simulink model "chaser_target_slosh"  (R2024a)
settings: Solver=VariableStepAuto  StartTime=0.0  StopTime=10.0  RelTol=1e-3
values from neighbouring files (symbols this model uses):
  dispslosh = 0.2    [main.m]
undefined symbols (not defined in the file or in its folder): chaser, InvDyn, KIN, reaction_wheels, slosh, solar_panel_big_reduced_FEM, solar_panel_target_reduced_FEM, target, ureal, uss, wn_big, wn_target
libraries: RCTblocks x54, SDTlibV1 x44
(part 1 of 3)
settings Model: Creator=T.FORMOSA  LastModifiedBy=r.de-oliveira
settings SolverCC: AlgebraicLoopSolver=TrustRegion
settings DebuggingCC: AlgebraicLoopMsg=none  UnconnectedInputMsg=warning  UnconnectedOutputMsg=warning  UnconnectedLineMsg=warning  ArithmeticOperatorsInVariantConditions=warning
settings ModelReferenceCC: EnableRefExpFcnMdlSchedulingChecks=on
settings SFSimCC: CustomCodeUndefinedFunction=UseInterfaceOnly
settings RTWCC: GPUComputeCapability=3.5  DLArmComputeVersion=19.05

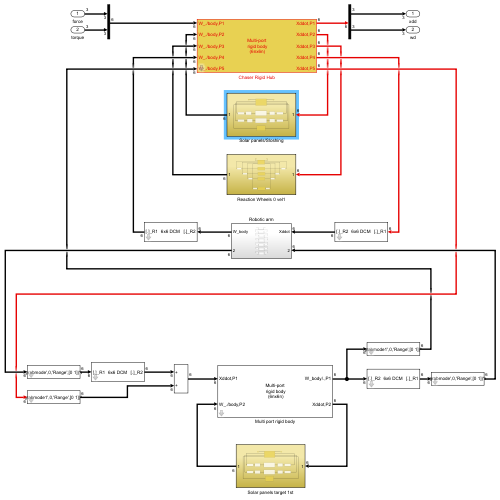
[thumbnail: Simulink's stored preview of the top-level diagram]
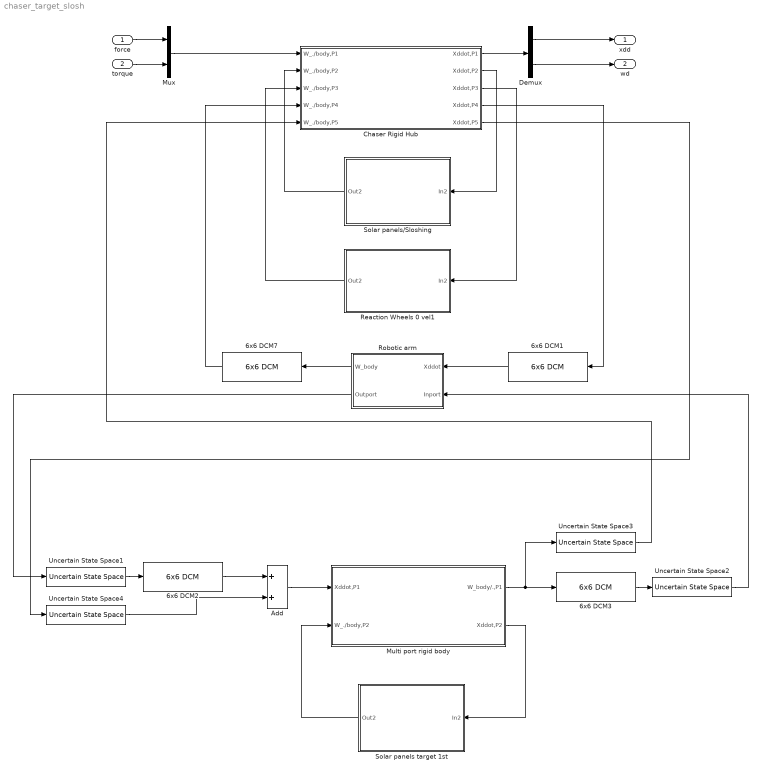
== system chaser_target_slosh ==
  force : Inport
  torque : Inport  Port=2
  6x6 DCM1 : SDTlibV1/3//6 dof DCM/6x6 DCM  rot=[-1 0 0;0 1 0;0 0 -1]  transp=on
      settings: SourceProductName=SDTlib
  6x6 DCM2 : SDTlibV1/3//6 dof DCM/6x6 DCM  rot=[0 1 0;1 0 0;0 0 -1]  transp=on
      settings: SourceProductName=SDTlib
  6x6 DCM3 : SDTlibV1/3//6 dof DCM/6x6 DCM  rot=[0 1 0;1 0 0;0 0 -1]  transp=off
      settings: SourceProductName=SDTlib
  6x6 DCM7 : SDTlibV1/3//6 dof DCM/6x6 DCM  rot=[-1 0 0;0 1 0;0 0 -1]  transp=off
      settings: SourceProductName=SDTlib
  Add : Sum
  Chaser Rigid Hub : Subsystem  mask(Multi-port rigid body (6nx6n)){m=chaser.rigidhub.wetmass, Ig=chaser.rigidhub.inertias, OG=[0;0;0], n=5, numinv=none, OP1=[0;0;0], OP2=[0;0;0], OP3=[0;0;0], OP4=[chaser.rigidhub.length/2*1.37;0;-chaser.rigidhub.height/2-0.01/2], OP5=[-1.8503e-1;-1.37618e-10;-6.3520e-1]}
      mask prompts: m "Mass (Kg)"; Ig "Inertia (at G, Kg m^2)"; OG "OG (3x1 vector, m)"; n "Number of ports"; numinv "Port to be inverted"; OP1 "OP1 (3x1 vector, m)"; OP2 "OP2 (3x1 vector, m)"; OP3 "OP3 (3x1 vector, m)"; OP4 "OP4 (3x1 vector, m)"; OP5 "OP5 (3x1 vector,m)"
      mask help:
      | 6nx6n inverse dynamic model between:
      |    *  wrenches applied to this body at the given n points,
      |    * acceleration twiists at he n given points.
      |
      | The 6x6 channel asociated to a single given point can be inverted
      mask init:
      | MultiPortRigidBody
      mask Help: web('Docmultiportrigidbody.html')
      mask TypeOptions n: 1 | 2 | 3 | 4 | 5
      mask TypeOptions numinv: none | 1 | 2 | 3 | 4 | 5
      mask DialogControl Control1 Prompt: Inverse Dynamic model of a rigid body at n given points (ports):
      mask DialogControl Control2 Prompt: 6nx6n transfer between wrenches applied at the n points and accelaretion twists at these points
      mask DialogControl Control3 Prompt: 0: the reference point
      mask DialogControl Control4 Prompt: G: the center of mass
      mask DialogControl Control5 Prompt: Pi (i=1:n): the n given connection points (n<6).
      mask DialogControl Control6 Prompt: All parameters are expressed in the body frame.
      mask DialogControl Control7 Prompt: Each parameter can be an uncertain parameter declared with "ureal"
      mask DialogControl Control8 Prompt: The 6x6 channel associated to one port can be inverted: then the input of this channel is the acceleration twist imposed at this point and the output is the wrench applied by this body.
      mask DialogControl ParameterGroupVar Prompt: Main parameters
      mask DialogControl port1 Prompt: Port #1
      mask DialogControl port2 Prompt: #2
      mask DialogControl port3 Prompt: #3
      mask DialogControl port4 Prompt: #4
      mask DialogControl port5 Prompt: #5
      mask Display:
      | disp('Multi-port\n rigid body\n (6nx6n)')
      | if n==1,
      |     if numinv-1==1,
      |         port_label('input', 1,'Xddot,P')
      |         port_label('output',1,'W_body/.,P')
      |     else
      |         port_label('input', 1,'W_./body,P')
      |         port_label('output',1,'Xddot,P')
      |     end
      | else
      |     for ii=1:n
      |         if numinv==ii+1,
      |             port_label('output',ii,['W_body/.,P',num2str(ii)])
      |             port_label('input', ii,['Xddot,P',num2str(ii)])
      |         else
      |             port_label('input', ii,['W_./body,P',num2str(ii)])
      |             port_label('output',ii,['Xddot,P',num2str(ii)])
      |         end
      |     end
      | end
  Demux : Demux  Outputs=[3 3]
  Multi port rigid body : Subsystem  mask(Multi-port rigid body (6nx6n)){m=target.rigidhub.wetmass_SDT, Ig=target.rigidhub.inertias_SDT, OG=[0;0;0], n=2, numinv=1, OP1=[-chaser.rigidhub.length*0.7/2;0;0]*ureal('grabmode',0,'Range',[0 1]), OP2=[0;0;0], OP3=[ureal('P3_y',1,'percent',10);0;0], OP4=[0;0;0], OP5=[0;0;0]}
      mask prompts: m "Mass (Kg)"; Ig "Inertia (at G, Kg m^2)"; OG "OG (3x1 vector, m)"; n "Number of ports"; numinv "Port to be inverted"; OP1 "OP1 (3x1 vector, m)"; OP2 "OP2 (3x1 vector, m)"; OP3 "OP3 (3x1 vector, m)"; OP4 "OP4 (3x1 vector, m)"; OP5 "OP5 (3x1 vector,m)"
      mask help:
      | 6nx6n dynamic model of a rigid body at n given points (ports) between wrenches applied at the n points (input) and acceleration twists at these points (output).
      |
      | 0: the reference point
      | G: the center of mass
      | Pi (i=1:n): the n given connection points (n<6).
      |
      | All parameters are expressed in the body frame.
      | Each parameter can be an uncertain parameter declared with "ureal"
      |
      | The 6x6 channel associated to one port can be inverted: then the input of this channel is the acceleration twist imposed at this point and the output is the wrench applied by this body.
      mask init:
      | MultiPortRigidBody
      mask Help: web('Docmultiportrigidbody.html')
      mask TypeOptions n: 1 | 2 | 3 | 4 | 5
      mask TypeOptions numinv: none | 1 | 2 | 3 | 4 | 5
      mask DialogControl ParameterGroupVar Prompt: Main parameters
      mask DialogControl port1 Prompt: Port #1
      mask DialogControl port2 Prompt: #2
      mask DialogControl port3 Prompt: #3
      mask DialogControl port4 Prompt: #4
      mask DialogControl port5 Prompt: #5
      mask Display:
      | disp('Multi-port\n rigid body\n (6nx6n)')
      | if n==1,
      |     if numinv-1==1,
      |         port_label('input', 1,'Xddot,P')
      |         port_label('output',1,'W_body/.,P')
      |     else
      |         port_label('input', 1,'W_./body,P')
      |         port_label('output',1,'Xddot,P')
      |     end
      | else
      |     for ii=1:n
      |         if numinv==ii+1,
      |             port_label('output',ii,['W_body/.,P',num2str(ii)])
      |             port_label('input', ii,['Xddot,P',num2str(ii)])
      |         else
      |             port_label('input', ii,['W_./body,P',num2str(ii)])
      |             port_label('output',ii,['Xddot,P',num2str(ii)])
      |         end
      |     end
      | end
  Mux : Mux  Inputs=[3 3]
  Reaction Wheels 0 vel1 : Subsystem
  Robotic arm : Subsystem
  Solar panels target 1st : Subsystem
  Solar panels/Sloshing : Subsystem
  Uncertain State Space1 : RCTblocks/Uncertain State Space  Tag=USS  USystem=ureal('grabmode',0,'Range',[0 1])*eye(6)  UValue=[]  X0=[]  uX0=[]
  Uncertain State Space2 : RCTblocks/Uncertain State Space  Tag=USS  USystem=ureal('grabmode',0,'Range',[0 1])*eye(6)  UValue=[]  X0=[]  uX0=[]
  Uncertain State Space3 : RCTblocks/Uncertain State Space  Tag=USS  USystem=ureal('grabmode1',0,'Range',[0 1])*eye(6)  UValue=[]  X0=[]  uX0=[]
  Uncertain State Space4 : RCTblocks/Uncertain State Space  Tag=USS  USystem=ureal('grabmode1',0,'Range',[0 1])*eye(6)  UValue=[]  X0=[]  uX0=[]
  xdd : Outport
  wd : Outport  Port=2
  wires:
  Reaction Wheels 0 vel1/1(Out2) -> Chaser Rigid Hub/3(W_./body,P3)
  Solar panels/Sloshing/1(Out2) -> Chaser Rigid Hub/2(W_./body,P2)
  Chaser Rigid Hub/1(Xddot,P1) -> Demux/1
  torque/1 -> Mux/2
  force/1 -> Mux/1
  Demux/1 -> xdd/1
  Chaser Rigid Hub/2(Xddot,P2) -> Solar panels/Sloshing/1(In2)
  Robotic arm/1(W_body) -> 6x6 DCM7/1
  6x6 DCM1/1 -> Robotic arm/1(Xddot)
  6x6 DCM7/1 -> Chaser Rigid Hub/4(W_./body,P4)
  6x6 DCM3/1 -> Uncertain State Space2/1
  Uncertain State Space1/1 -> 6x6 DCM2/1
  Uncertain State Space4/1 -> Add/2
  Add/1 -> Multi port rigid body/1(Xddot,P1)
  Multi port rigid body/2(Xddot,P2) -> Solar panels target 1st/1(In2)
  Solar panels target 1st/1(Out2) -> Multi port rigid body/2(W_./body,P2)
  6x6 DCM2/1 -> Add/1
  Chaser Rigid Hub/3(Xddot,P3) -> Reaction Wheels 0 vel1/1(In2)
  Chaser Rigid Hub/4(Xddot,P4) -> 6x6 DCM1/1
  Chaser Rigid Hub/5(Xddot,P5) -> Uncertain State Space4/1
  Uncertain State Space3/1 -> Chaser Rigid Hub/5(W_./body,P5)
  Robotic arm/2(Outport) -> Uncertain State Space1/1
  Uncertain State Space2/1 -> Robotic arm/2(Inport)
  Mux/1 -> Chaser Rigid Hub/1(W_./body,P1)
  Demux/2 -> wd/1
  Multi port rigid body/1(W_body/.,P1) -> Uncertain State Space3/1, 6x6 DCM3/1

== system chaser_target_slosh/Chaser Rigid Hub ==
  W_./body,P1 : Inport  PortDimensions=6
  W_./body,P2 : Inport  Port=2  PortDimensions=6
  W_./body,P3 : Inport  Port=3  PortDimensions=6
  W_./body,P4 : Inport  Port=4  PortDimensions=6
  W_./body,P5 : Inport  Port=5  PortDimensions=6
  Demux : Demux  Outputs=[6 6 6 6 6]
  Gain : RCTblocks/Uncertain State Space  Tag=USS  USystem=uss(InvDyn)  UValue=[]  X0=[]  uX0=[]
  Mux : Mux  Inputs=[6 6 6 6 6]
  Xddot,P1 : Outport
  Xddot,P2 : Outport  Port=2
  Xddot,P3 : Outport  Port=3
  Xddot,P4 : Outport  Port=4
  Xddot,P5 : Outport  Port=5
  wires:
  Mux/1 -> Gain/1
  Gain/1 -> Demux/1
  W_./body,P1/1 -> Mux/1
  Demux/1 -> Xddot,P1/1
  W_./body,P2/1 -> Mux/2
  Demux/2 -> Xddot,P2/1
  W_./body,P3/1 -> Mux/3
  Demux/3 -> Xddot,P3/1
  W_./body,P4/1 -> Mux/4
  Demux/4 -> Xddot,P4/1
  W_./body,P5/1 -> Mux/5
  Demux/5 -> Xddot,P5/1

== system chaser_target_slosh/Multi port rigid body ==
  Xddot,P1 : Inport  PortDimensions=6
  W_./body,P2 : Inport  Port=2  PortDimensions=6
  Demux : Demux  Outputs=[6 6]
  Gain : RCTblocks/Uncertain State Space  Tag=USS  USystem=uss(InvDyn)  UValue=[]  X0=[]  uX0=[]
  Mux : Mux  Inputs=[6 6]
  W_body/.,P1 : Outport
  Xddot,P2 : Outport  Port=2
  wires:
  Mux/1 -> Gain/1
  Gain/1 -> Demux/1
  Xddot,P1/1 -> Mux/1
  Demux/1 -> W_body/.,P1/1
  W_./body,P2/1 -> Mux/2
  Demux/2 -> Xddot,P2/1

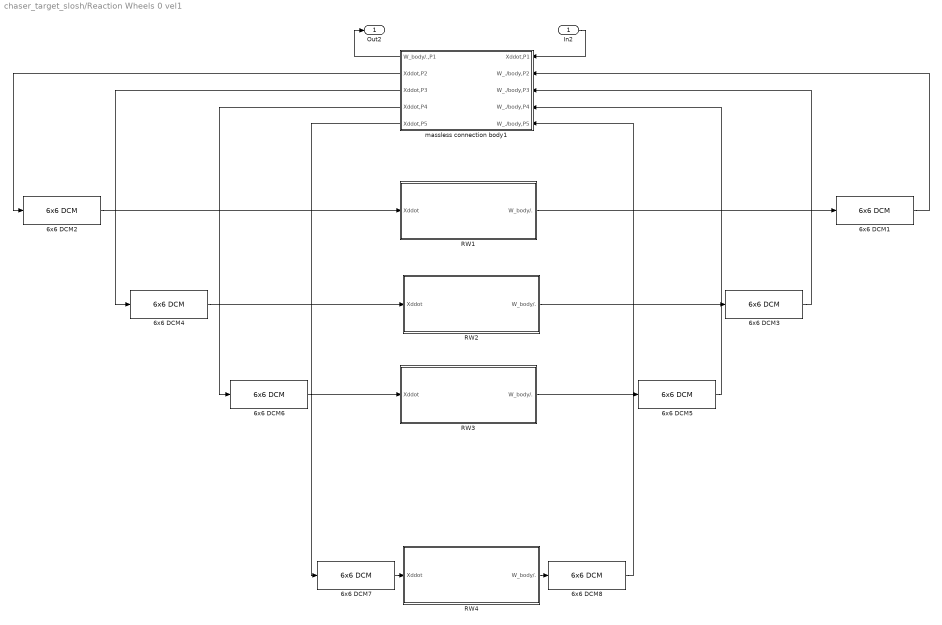
== system chaser_target_slosh/Reaction Wheels 0 vel1 ==
  In2 : Inport
  6x6 DCM1 : SDTlibV1/3//6 dof DCM/6x6 DCM  rot=chaser.GNC.control.reaction_wheels.DCM(:, :, 1)  transp=off
      settings: SourceProductName=SDTlib
  6x6 DCM2 : SDTlibV1/3//6 dof DCM/6x6 DCM  rot=chaser.GNC.control.reaction_wheels.DCM(:, :, 1)  transp=on
      settings: SourceProductName=SDTlib
  6x6 DCM3 : SDTlibV1/3//6 dof DCM/6x6 DCM  rot=chaser.GNC.control.reaction_wheels.DCM(:, :, 2)  transp=off
      settings: SourceProductName=SDTlib
  6x6 DCM4 : SDTlibV1/3//6 dof DCM/6x6 DCM  rot=chaser.GNC.control.reaction_wheels.DCM(:, :, 2)  transp=on
      settings: SourceProductName=SDTlib
  6x6 DCM5 : SDTlibV1/3//6 dof DCM/6x6 DCM  rot=chaser.GNC.control.reaction_wheels.DCM(:, :, 3)  transp=off
      settings: SourceProductName=SDTlib
  6x6 DCM6 : SDTlibV1/3//6 dof DCM/6x6 DCM  rot=chaser.GNC.control.reaction_wheels.DCM(:, :, 3)  transp=on
      settings: SourceProductName=SDTlib
  6x6 DCM7 : SDTlibV1/3//6 dof DCM/6x6 DCM  rot=chaser.GNC.control.reaction_wheels.DCM(:, :, 4)  transp=on
      settings: SourceProductName=SDTlib
  6x6 DCM8 : SDTlibV1/3//6 dof DCM/6x6 DCM  rot=chaser.GNC.control.reaction_wheels.DCM(:, :, 4)  transp=off
      settings: SourceProductName=SDTlib
  RW1 : Subsystem  AncestorBlock=SDTlibV1/6 dof bodies/1 port spinning wheel  mask(One-port spinning wheel (6x6)){ra=[0;0;1], m=chaser.reactionwheels.mass, Iw=chaser.reactionwheels.axialinertia, Ir=chaser.reactionwheels.radialinertia, OG=[0;0;0], OP=[0;0;0], Omega=reaction_wheels.initial_w_SDT(1)}
      mask prompts: ra "Wheel axis (3x1 vector)"; m "Wheel mass (Kg)"; Iw "Wheel axial Inertia  (at G, Kgm^2)"; Ir "Wheel radial inertia (at G, Kgm^2)"; OG "OG (3x1 vector, m)"; OP "OP (3x1 vector, m)"; Omega "spinning rate (rd/s)"
      mask help:
      | Dynamic model of an onboard angular momentum (spinning wheel) at point P (connection point with a parent body):
      | 6x6 transfer between accelaretion twist at P and wrench applied by this body at P.
      | 0: the reference point
      | G: the center of the wheel
      | P: the connection point
      |
      | All parameters are expressed in the (inherit) body frame.
      | Only the spinning rate can be an uncertain parameter declared with "ureal"
      mask init:
      | pass=ra2DCMi(ra);
      | Tau_GP=kinematic_model(OG,OP);
      mask Help: web('DocMomentum.html')
      mask DialogControl ParameterGroupVar Prompt: Main parameters
      mask Display:
      | disp('One-port\n angular momemtum\n (6x6)')
      | port_label('input', 1, 'Xddot')
      | port_label('output', 1, 'W_body/.')
  RW2 : Subsystem  AncestorBlock=SDTlibV1/6 dof bodies/1 port spinning wheel  mask(One-port spinning wheel (6x6)){ra=[0;0;1], m=chaser.reactionwheels.mass, Iw=chaser.reactionwheels.axialinertia, Ir=chaser.reactionwheels.radialinertia, OG=[0;0;0], OP=[0;0;0], Omega=reaction_wheels.initial_w_SDT(2)}
      mask prompts: ra "Wheel axis (3x1 vector)"; m "Wheel mass (Kg)"; Iw "Wheel axial Inertia  (at G, Kgm^2)"; Ir "Wheel radial inertia (at G, Kgm^2)"; OG "OG (3x1 vector, m)"; OP "OP (3x1 vector, m)"; Omega "spinning rate (rd/s)"
      mask help:
      | Dynamic model of an onboard angular momentum (spinning wheel) at point P (connection point with a parent body):
      | 6x6 transfer between accelaretion twist at P and wrench applied by this body at P.
      | 0: the reference point
      | G: the center of the wheel
      | P: the connection point
      |
      | All parameters are expressed in the (inherit) body frame.
      | Only the spinning rate can be an uncertain parameter declared with "ureal"
      mask init:
      | pass=ra2DCMi(ra);
      | Tau_GP=kinematic_model(OG,OP);
      mask Help: web('DocMomentum.html')
      mask DialogControl ParameterGroupVar Prompt: Main parameters
      mask Display:
      | disp('One-port\n angular momemtum\n (6x6)')
      | port_label('input', 1, 'Xddot')
      | port_label('output', 1, 'W_body/.')
  RW3 : Subsystem  AncestorBlock=SDTlibV1/6 dof bodies/1 port spinning wheel  mask(One-port spinning wheel (6x6)){ra=[0;0;1], m=chaser.reactionwheels.mass, Iw=chaser.reactionwheels.axialinertia, Ir=chaser.reactionwheels.radialinertia, OG=[0;0;0], OP=[0;0;0], Omega=reaction_wheels.initial_w_SDT(3)}
      mask prompts: ra "Wheel axis (3x1 vector)"; m "Wheel mass (Kg)"; Iw "Wheel axial Inertia  (at G, Kgm^2)"; Ir "Wheel radial inertia (at G, Kgm^2)"; OG "OG (3x1 vector, m)"; OP "OP (3x1 vector, m)"; Omega "spinning rate (rd/s)"
      mask help:
      | Dynamic model of an onboard angular momentum (spinning wheel) at point P (connection point with a parent body):
      | 6x6 transfer between accelaretion twist at P and wrench applied by this body at P.
      | 0: the reference point
      | G: the center of the wheel
      | P: the connection point
      |
      | All parameters are expressed in the (inherit) body frame.
      | Only the spinning rate can be an uncertain parameter declared with "ureal"
      mask init:
      | pass=ra2DCMi(ra);
      | Tau_GP=kinematic_model(OG,OP);
      mask Help: web('DocMomentum.html')
      mask DialogControl ParameterGroupVar Prompt: Main parameters
      mask Display:
      | disp('One-port\n angular momemtum\n (6x6)')
      | port_label('input', 1, 'Xddot')
      | port_label('output', 1, 'W_body/.')
  RW4 : Subsystem  AncestorBlock=SDTlibV1/6 dof bodies/1 port spinning wheel  mask(One-port spinning wheel (6x6)){ra=[0;0;1], m=chaser.reactionwheels.mass, Iw=chaser.reactionwheels.axialinertia, Ir=chaser.reactionwheels.radialinertia, OG=[0;0;0], OP=[0;0;0], Omega=reaction_wheels.initial_w_SDT(4)}
      mask prompts: ra "Wheel axis (3x1 vector)"; m "Wheel mass (Kg)"; Iw "Wheel axial Inertia  (at G, Kgm^2)"; Ir "Wheel radial inertia (at G, Kgm^2)"; OG "OG (3x1 vector, m)"; OP "OP (3x1 vector, m)"; Omega "spinning rate (rd/s)"
      mask help:
      | Dynamic model of an onboard angular momentum (spinning wheel) at point P (connection point with a parent body):
      | 6x6 transfer between accelaretion twist at P and wrench applied by this body at P.
      | 0: the reference point
      | G: the center of the wheel
      | P: the connection point
      |
      | All parameters are expressed in the (inherit) body frame.
      | Only the spinning rate can be an uncertain parameter declared with "ureal"
      mask init:
      | pass=ra2DCMi(ra);
      | Tau_GP=kinematic_model(OG,OP);
      mask Help: web('DocMomentum.html')
      mask DialogControl ParameterGroupVar Prompt: Main parameters
      mask Display:
      | disp('One-port\n angular momemtum\n (6x6)')
      | port_label('input', 1, 'Xddot')
      | port_label('output', 1, 'W_body/.')
  massless connection body1 : Subsystem  mask(Massless multi_port (6nx6n)){n=5, numinv=1, OP1=[0;0;0], OP2=chaser.GNC.control.reaction_wheels.positions(:,1), OP3=chaser.GNC.control.reaction_wheels.positions(:,2), OP4=chaser.GNC.control.reaction_wheels.positions(:,3), OP5=chaser.GNC.control.reaction_wheels.positions(:,4), OP6=[0;0;0], OP7=[0;0;0]}
      mask prompts: n "Number of ports"; numinv "Port (point) Pj: j="; OP1 "OP1 (3x1 vector, m)"; OP2 "OP2 (3x1 vector, m)"; OP3 "OP3 (3x1 vector, m)"; OP4 "OP4 (3x1 vector, m)"; OP5 "OP5 (3x1 vector,m)"; OP6 "OP6 (3x1 vector,m)"; OP7 "OP7 (3x1 vector,m)"
      mask help:
      | Massless body to transport wrenches and acceleration twists:
      | 6nx6n gain from:
      |  * the acceleration twist at one point Pj; i.e. the parent port,
      |  * the wrenches applied to this massless body at the n-1 points Pi (i=1,..n, except j); i.e. the child ports
      | to:
      |  * the wrench applied at point Pj by this massless body,
      |  * the accelaretion twists at the other n-1  points Pi (i=1,..n, except j).
      |
      | 0: the reference point
      | Pi (i=1:n): the n given connection points or ports (1<n<8).
      |
      | All parameters are expressed in the body frame.
      | Each parameter can be an uncertain parameter declared with "ureal"
      mask init:
      | MasslessConnectionBody
      mask Help: web('DocMassLessBody.html')
      mask TypeOptions n: 2 | 3 | 4 | 5 | 6 | 7
      mask TypeOptions numinv: 1 | 2 | 3 | 4 | 5 | 6 | 7
      mask DialogControl ParameterGroupVar Prompt: Main parameters
      mask DialogControl port1 Prompt: Port #1
      mask DialogControl port2 Prompt: #2
      mask DialogControl port3 Prompt: #3
      mask DialogControl port4 Prompt: #4
      mask DialogControl port5 Prompt: #5
      mask DialogControl port6 Prompt: #6
      mask DialogControl port7 Prompt: #7
      mask Display:
      | disp('Massless\n connection body\n (6nx6n)')
      | for ii=1:n+1
      |     if numinv==ii,
      |         port_label('output',ii,['W_body/.,P',num2str(ii)])
      |         port_label('input', ii,['Xddot,P',num2str(ii)])
      |     else
      |         port_label('input', ii,['W_./body,P',num2str(ii)])
      |         port_label('output',ii,['Xddot,P',num2str(ii)])
      |     end
      | end
  Out2 : Outport
  wires:
  massless connection body1/1(W_body/.,P1) -> Out2/1
  massless connection body1/2(Xddot,P2) -> 6x6 DCM2/1
  In2/1 -> massless connection body1/1(Xddot,P1)
  RW2/1(W_body/.) -> 6x6 DCM3/1
  massless connection body1/3(Xddot,P3) -> 6x6 DCM4/1
  massless connection body1/4(Xddot,P4) -> 6x6 DCM6/1
  RW3/1(W_body/.) -> 6x6 DCM5/1
  massless connection body1/5(Xddot,P5) -> 6x6 DCM7/1
  RW4/1(W_body/.) -> 6x6 DCM8/1
  6x6 DCM1/1 -> massless connection body1/2(W_./body,P2)
  6x6 DCM2/1 -> RW1/1(Xddot)
  6x6 DCM3/1 -> massless connection body1/3(W_./body,P3)
  6x6 DCM4/1 -> RW2/1(Xddot)
  6x6 DCM5/1 -> massless connection body1/4(W_./body,P4)
  6x6 DCM6/1 -> RW3/1(Xddot)
  6x6 DCM7/1 -> RW4/1(Xddot)
  6x6 DCM8/1 -> massless connection body1/5(W_./body,P5)
  RW1/1(W_body/.) -> 6x6 DCM1/1

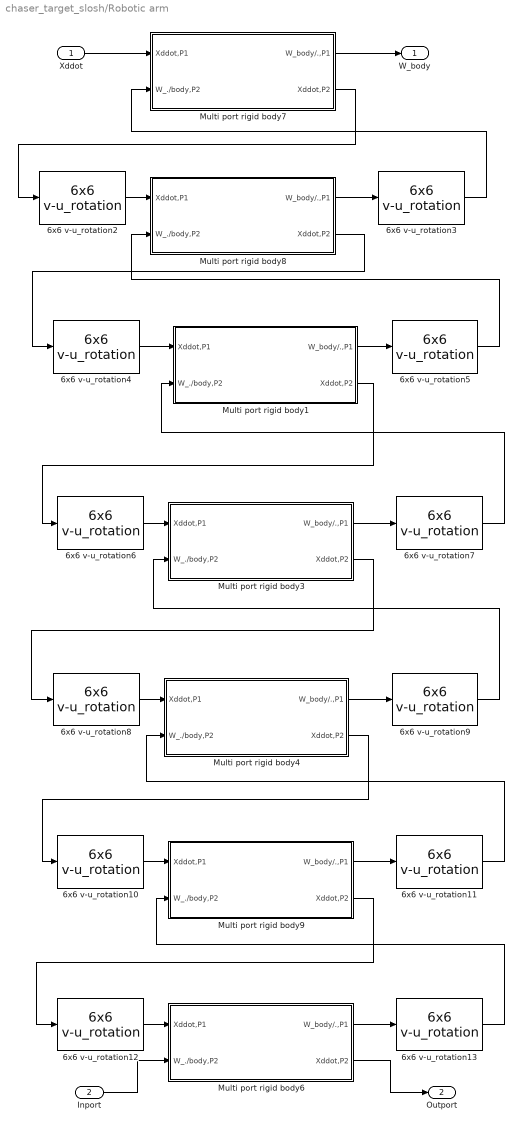
== system chaser_target_slosh/Robotic arm ==
  Xddot : Inport
  Inport : Inport  Port=2
  6x6 v-u_rotation10 : SDTlibV1/3//6 dof DCM/6x6 v-u_rotation  ra=[0;0;-1]  theta=ureal('theta5',0,'Range',[-pi pi])  transp=on
      settings: SourceProductName=SDTlib
  6x6 v-u_rotation11 : SDTlibV1/3//6 dof DCM/6x6 v-u_rotation  ra=[0;0;-1]  theta=ureal('theta5',0,'Range',[-pi pi])  transp=off
      settings: SourceProductName=SDTlib
  6x6 v-u_rotation12 : SDTlibV1/3//6 dof DCM/6x6 v-u_rotation  ra=[0;1;0]  theta=ureal('theta6',0,'Range',[-pi pi])  transp=on
      settings: SourceProductName=SDTlib
  6x6 v-u_rotation13 : SDTlibV1/3//6 dof DCM/6x6 v-u_rotation  ra=[0;1;0]  theta=ureal('theta6',0,'Range',[-pi pi])  transp=off
      settings: SourceProductName=SDTlib
  6x6 v-u_rotation2 : SDTlibV1/3//6 dof DCM/6x6 v-u_rotation  ra=[0;0;1]  theta=ureal('theta1',0,'Range',[-pi pi])  transp=on
      settings: SourceProductName=SDTlib
  6x6 v-u_rotation3 : SDTlibV1/3//6 dof DCM/6x6 v-u_rotation  ra=[0;0;1]  theta=ureal('theta1',0,'Range',[-pi pi])  transp=off
      settings: SourceProductName=SDTlib
  6x6 v-u_rotation4 : SDTlibV1/3//6 dof DCM/6x6 v-u_rotation  ra=[0;1;0]  theta=ureal('theta2',0,'Range',[-pi pi])  transp=on
      settings: SourceProductName=SDTlib
  6x6 v-u_rotation5 : SDTlibV1/3//6 dof DCM/6x6 v-u_rotation  ra=[0;1;0]  theta=ureal('theta2',0,'Range',[-pi pi])  transp=off
      settings: SourceProductName=SDTlib
  6x6 v-u_rotation6 : SDTlibV1/3//6 dof DCM/6x6 v-u_rotation  ra=[0;1;0]  theta=ureal('theta3',0,'Range',[-pi pi])  transp=on
      settings: SourceProductName=SDTlib
  6x6 v-u_rotation7 : SDTlibV1/3//6 dof DCM/6x6 v-u_rotation  ra=[0;1;0]  theta=ureal('theta3',0,'Range',[-pi pi])  transp=off
      settings: SourceProductName=SDTlib
  6x6 v-u_rotation8 : SDTlibV1/3//6 dof DCM/6x6 v-u_rotation  ra=[0;1;0]  theta=ureal('theta4',0,'Range',[-pi pi])  transp=on
      settings: SourceProductName=SDTlib
  6x6 v-u_rotation9 : SDTlibV1/3//6 dof DCM/6x6 v-u_rotation  ra=[0;1;0]  theta=ureal('theta4',0,'Range',[-pi pi])  transp=off
      settings: SourceProductName=SDTlib
  Multi port rigid body1 : Subsystem  mask(Multi-port rigid body (6nx6n)){m=8.393000000000001, Ig=[0.0151074 0 0;0 0.22689067591 0;0 0 0.22689067591], OG=[0.28;0;0], n=2, numinv=1, OP1=[0;0;0], OP2=[0.425; -0.1197; 0], OP3=[0;0;0], OP4=[0;0;0], OP5=[0;0;0]}
      mask prompts: m "Mass (Kg)"; Ig "Inertia (at G, Kg m^2)"; OG "OG (3x1 vector, m)"; n "Number of ports"; numinv "Port to be inverted"; OP1 "OP1 (3x1 vector, m)"; OP2 "OP2 (3x1 vector, m)"; OP3 "OP3 (3x1 vector, m)"; OP4 "OP4 (3x1 vector, m)"; OP5 "OP5 (3x1 vector,m)"
      mask help:
      | 6nx6n dynamic model of a rigid body at n given points (ports) between wrenches applied at the n points (input) and acceleration twists at these points (output).
      |
      | 0: the reference point
      | G: the center of mass
      | Pi (i=1:n): the n given connection points (n<6).
      |
      | All parameters are expressed in the body frame.
      | Each parameter can be an uncertain parameter declared with "ureal"
      |
      | The 6x6 channel associated to one port can be inverted: then the input of this channel is the acceleration twist imposed at this point and the output is the wrench applied by this body.
      mask init:
      | MultiPortRigidBody
      mask Help: web('Docmultiportrigidbody.html')
      mask TypeOptions n: 1 | 2 | 3 | 4 | 5
      mask TypeOptions numinv: none | 1 | 2 | 3 | 4 | 5
      mask DialogControl ParameterGroupVar Prompt: Main parameters
      mask DialogControl port1 Prompt: Port #1
      mask DialogControl port2 Prompt: #2
      mask DialogControl port3 Prompt: #3
      mask DialogControl port4 Prompt: #4
      mask DialogControl port5 Prompt: #5
      mask Display:
      | disp('Multi-port\n rigid body\n (6nx6n)')
      | if n==1,
      |     if numinv-1==1,
      |         port_label('input', 1,'Xddot,P')
      |         port_label('output',1,'W_body/.,P')
      |     else
      |         port_label('input', 1,'W_./body,P')
      |         port_label('output',1,'Xddot,P')
      |     end
      | else
      |     for ii=1:n
      |         if numinv==ii+1,
      |             port_label('output',ii,['W_body/.,P',num2str(ii)])
      |             port_label('input', ii,['Xddot,P',num2str(ii)])
      |         else
      |             port_label('input', ii,['W_./body,P',num2str(ii)])
      |             port_label('output',ii,['Xddot,P',num2str(ii)])
      |         end
      |     end
      | end
  Multi port rigid body3 : Subsystem  mask(Multi-port rigid body (6nx6n)){m=2.275, Ig=[0.004095 0 0;0 0.049443313556 0;0 0 0.049443313556], OG=[0.25;0;0], n=2, numinv=1, OP1=[0;0;0], OP2=[0.39225; 0; 0], OP3=[0;0;0], OP4=[0;0;0], OP5=[0;0;0]}
      mask prompts: m "Mass (Kg)"; Ig "Inertia (at G, Kg m^2)"; OG "OG (3x1 vector, m)"; n "Number of ports"; numinv "Port to be inverted"; OP1 "OP1 (3x1 vector, m)"; OP2 "OP2 (3x1 vector, m)"; OP3 "OP3 (3x1 vector, m)"; OP4 "OP4 (3x1 vector, m)"; OP5 "OP5 (3x1 vector,m)"
      mask help:
      | 6nx6n dynamic model of a rigid body at n given points (ports) between wrenches applied at the n points (input) and acceleration twists at these points (output).
      |
      | 0: the reference point
      | G: the center of mass
      | Pi (i=1:n): the n given connection points (n<6).
      |
      | All parameters are expressed in the body frame.
      | Each parameter can be an uncertain parameter declared with "ureal"
      |
      | The 6x6 channel associated to one port can be inverted: then the input of this channel is the acceleration twist imposed at this point and the output is the wrench applied by this body.
      mask init:
      | MultiPortRigidBody
      mask Help: web('Docmultiportrigidbody.html')
      mask TypeOptions n: 1 | 2 | 3 | 4 | 5
      mask TypeOptions numinv: none | 1 | 2 | 3 | 4 | 5
      mask DialogControl ParameterGroupVar Prompt: Main parameters
      mask DialogControl port1 Prompt: Port #1
      mask DialogControl port2 Prompt: #2
      mask DialogControl port3 Prompt: #3
      mask DialogControl port4 Prompt: #4
      mask DialogControl port5 Prompt: #5
      mask Display:
      | disp('Multi-port\n rigid body\n (6nx6n)')
      | if n==1,
      |     if numinv-1==1,
      |         port_label('input', 1,'Xddot,P')
      |         port_label('output',1,'W_body/.,P')
      |     else
      |         port_label('input', 1,'W_./body,P')
      |         port_label('output',1,'Xddot,P')
      |     end
      | else
      |     for ii=1:n
      |         if numinv==ii+1,
      |             port_label('output',ii,['W_body/.,P',num2str(ii)])
      |             port_label('input', ii,['Xddot,P',num2str(ii)])
      |         else
      |             port_label('input', ii,['W_./body,P',num2str(ii)])
      |             port_label('output',ii,['Xddot,P',num2str(ii)])
      |         end
      |     end
      | end
  Multi port rigid body4 : Subsystem  mask(Multi-port rigid body (6nx6n)){m=1.219, Ig=[0.111172755531 0 0;0 0.111172755531 0;0 0 0.21942], OG=[0;0;0], n=2, numinv=1, OP1=[0;0;0], OP2=[0; 0.093; 0], OP3=[0;0;0], OP4=[0;0;0], OP5=[0;0;0]}
      mask prompts: m "Mass (Kg)"; Ig "Inertia (at G, Kg m^2)"; OG "OG (3x1 vector, m)"; n "Number of ports"; numinv "Port to be inverted"; OP1 "OP1 (3x1 vector, m)"; OP2 "OP2 (3x1 vector, m)"; OP3 "OP3 (3x1 vector, m)"; OP4 "OP4 (3x1 vector, m)"; OP5 "OP5 (3x1 vector,m)"
      mask help:
      | 6nx6n dynamic model of a rigid body at n given points (ports) between wrenches applied at the n points (input) and acceleration twists at these points (output).
      |
      | 0: the reference point
      | G: the center of mass
      | Pi (i=1:n): the n given connection points (n<6).
      |
      | All parameters are expressed in the body frame.
      | Each parameter can be an uncertain parameter declared with "ureal"
      |
      | The 6x6 channel associated to one port can be inverted: then the input of this channel is the acceleration twist imposed at this point and the output is the wrench applied by this body.
      mask init:
      | MultiPortRigidBody
      mask Help: web('Docmultiportrigidbody.html')
      mask TypeOptions n: 1 | 2 | 3 | 4 | 5
      mask TypeOptions numinv: none | 1 | 2 | 3 | 4 | 5
      mask DialogControl ParameterGroupVar Prompt: Main parameters
      mask DialogControl port1 Prompt: Port #1
      mask DialogControl port2 Prompt: #2
      mask DialogControl port3 Prompt: #3
      mask DialogControl port4 Prompt: #4
      mask DialogControl port5 Prompt: #5
      mask Display:
      | disp('Multi-port\n rigid body\n (6nx6n)')
      | if n==1,
      |     if numinv-1==1,
      |         port_label('input', 1,'Xddot,P')
      |         port_label('output',1,'W_body/.,P')
      |     else
      |         port_label('input', 1,'W_./body,P')
      |         port_label('output',1,'Xddot,P')
      |     end
      | else
      |     for ii=1:n
      |         if numinv==ii+1,
      |             port_label('output',ii,['W_body/.,P',num2str(ii)])
      |             port_label('input', ii,['Xddot,P',num2str(ii)])
      |         else
      |             port_label('input', ii,['W_./body,P',num2str(ii)])
      |             port_label('output',ii,['Xddot,P',num2str(ii)])
      |         end
      |     end
      | end
  Multi port rigid body6 : Subsystem  mask(Multi-port rigid body (6nx6n)){m=0.1879, Ig=[0.0171364731454 0 0;0 0.0171364731454 0;0 0 0.033822], OG=[0;0;0], n=2, numinv=1, OP1=[0;0;0], OP2=[0; 0.0823; 0], OP3=[0;0;0], OP4=[0;0;0], OP5=[0;0;0]}
      mask prompts: m "Mass (Kg)"; Ig "Inertia (at G, Kg m^2)"; OG "OG (3x1 vector, m)"; n "Number of ports"; numinv "Port to be inverted"; OP1 "OP1 (3x1 vector, m)"; OP2 "OP2 (3x1 vector, m)"; OP3 "OP3 (3x1 vector, m)"; OP4 "OP4 (3x1 vector, m)"; OP5 "OP5 (3x1 vector,m)"
      mask help:
      | 6nx6n dynamic model of a rigid body at n given points (ports) between wrenches applied at the n points (input) and acceleration twists at these points (output).
      |
      | 0: the reference point
      | G: the center of mass
      | Pi (i=1:n): the n given connection points (n<6).
      |
      | All parameters are expressed in the body frame.
      | Each parameter can be an uncertain parameter declared with "ureal"
      |
      | The 6x6 channel associated to one port can be inverted: then the input of this channel is the acceleration twist imposed at this point and the output is the wrench applied by this body.
      mask init:
      | MultiPortRigidBody
      mask Help: web('Docmultiportrigidbody.html')
      mask TypeOptions n: 1 | 2 | 3 | 4 | 5
      mask TypeOptions numinv: none | 1 | 2 | 3 | 4 | 5
      mask DialogControl ParameterGroupVar Prompt: Main parameters
      mask DialogControl port1 Prompt: Port #1
      mask DialogControl port2 Prompt: #2
      mask DialogControl port3 Prompt: #3
      mask DialogControl port4 Prompt: #4
      mask DialogControl port5 Prompt: #5
      mask Display:
      | disp('Multi-port\n rigid body\n (6nx6n)')
      | if n==1,
      |     if numinv-1==1,
      |         port_label('input', 1,'Xddot,P')
      |         port_label('output',1,'W_body/.,P')
      |     else
      |         port_label('input', 1,'W_./body,P')
      |         port_label('output',1,'Xddot,P')
      |     end
      | else
      |     for ii=1:n
      |         if numinv==ii+1,
      |             port_label('output',ii,['W_body/.,P',num2str(ii)])
      |             port_label('input', ii,['Xddot,P',num2str(ii)])
      |         else
      |             port_label('input', ii,['W_./body,P',num2str(ii)])
      |             port_label('output',ii,['Xddot,P',num2str(ii)])
      |         end
      |     end
      | end
  Multi port rigid body7 : Subsystem  mask(Multi-port rigid body (6nx6n)){m=4, Ig=[0.00443333156 0 0; 0 0.00443333156 0; 0 0 0.0072], OG=[0;0;0], n=2, numinv=1, OP1=[0;0;0], OP2=[0;0;0.089159], OP3=[0;0;0], OP4=[0;0;0], OP5=[0;0;0]}
      mask prompts: m "Mass (Kg)"; Ig "Inertia (at G, Kg m^2)"; OG "OG (3x1 vector, m)"; n "Number of ports"; numinv "Port to be inverted"; OP1 "OP1 (3x1 vector, m)"; OP2 "OP2 (3x1 vector, m)"; OP3 "OP3 (3x1 vector, m)"; OP4 "OP4 (3x1 vector, m)"; OP5 "OP5 (3x1 vector,m)"
      mask help:
      | 6nx6n dynamic model of a rigid body at n given points (ports) between wrenches applied at the n points (input) and acceleration twists at these points (output).
      |
      | 0: the reference point
      | G: the center of mass
      | Pi (i=1:n): the n given connection points (n<6).
      |
      | All parameters are expressed in the body frame.
      | Each parameter can be an uncertain parameter declared with "ureal"
      |
      | The 6x6 channel associated to one port can be inverted: then the input of this channel is the acceleration twist imposed at this point and the output is the wrench applied by this body.
      mask init:
      | MultiPortRigidBody
      mask Help: web('Docmultiportrigidbody.html')
      mask TypeOptions n: 1 | 2 | 3 | 4 | 5
      mask TypeOptions numinv: none | 1 | 2 | 3 | 4 | 5
      mask DialogControl ParameterGroupVar Prompt: Main parameters
      mask DialogControl port1 Prompt: Port #1
      mask DialogControl port2 Prompt: #2
      mask DialogControl port3 Prompt: #3
      mask DialogControl port4 Prompt: #4
      mask DialogControl port5 Prompt: #5
      mask Display:
      | disp('Multi-port\n rigid body\n (6nx6n)')
      | if n==1,
      |     if numinv-1==1,
      |         port_label('input', 1,'Xddot,P')
      |         port_label('output',1,'W_body/.,P')
      |     else
      |         port_label('input', 1,'W_./body,P')
      |         port_label('output',1,'Xddot,P')
      |     end
      | else
      |     for ii=1:n
      |         if numinv==ii+1,
      |             port_label('output',ii,['W_body/.,P',num2str(ii)])
      |             port_label('input', ii,['Xddot,P',num2str(ii)])
      |         else
      |             port_label('input', ii,['W_./body,P',num2str(ii)])
      |             port_label('output',ii,['Xddot,P',num2str(ii)])
      |         end
      |     end
      | end
  Multi port rigid body8 : Subsystem  mask(Multi-port rigid body (6nx6n)){m=3.7, Ig=[0.010267495893 0 0; 0 0.010267495893 0; 0 0 0.00666], OG=[0;0;0], n=2, numinv=1, OP1=[0;0;0], OP2=[0;0.13585;0], OP3=[0;0;0], OP4=[0;0;0], OP5=[0;0;0]}
      mask prompts: m "Mass (Kg)"; Ig "Inertia (at G, Kg m^2)"; OG "OG (3x1 vector, m)"; n "Number of ports"; numinv "Port to be inverted"; OP1 "OP1 (3x1 vector, m)"; OP2 "OP2 (3x1 vector, m)"; OP3 "OP3 (3x1 vector, m)"; OP4 "OP4 (3x1 vector, m)"; OP5 "OP5 (3x1 vector,m)"
      mask help:
      | 6nx6n dynamic model of a rigid body at n given points (ports) between wrenches applied at the n points (input) and acceleration twists at these points (output).
      |
      | 0: the reference point
      | G: the center of mass
      | Pi (i=1:n): the n given connection points (n<6).
      |
      | All parameters are expressed in the body frame.
      | Each parameter can be an uncertain parameter declared with "ureal"
      |
      | The 6x6 channel associated to one port can be inverted: then the input of this channel is the acceleration twist imposed at this point and the output is the wrench applied by this body.
      mask init:
      | MultiPortRigidBody
      mask Help: web('Docmultiportrigidbody.html')
      mask TypeOptions n: 1 | 2 | 3 | 4 | 5
      mask TypeOptions numinv: none | 1 | 2 | 3 | 4 | 5
      mask DialogControl ParameterGroupVar Prompt: Main parameters
      mask DialogControl port1 Prompt: Port #1
      mask DialogControl port2 Prompt: #2
      mask DialogControl port3 Prompt: #3
      mask DialogControl port4 Prompt: #4
      mask DialogControl port5 Prompt: #5
      mask Display:
      | disp('Multi-port\n rigid body\n (6nx6n)')
      | if n==1,
      |     if numinv-1==1,
      |         port_label('input', 1,'Xddot,P')
      |         port_label('output',1,'W_body/.,P')
      |     else
      |         port_label('input', 1,'W_./body,P')
      |         port_label('output',1,'Xddot,P')
      |     end
      | else
      |     for ii=1:n
      |         if numinv==ii+1,
      |             port_label('output',ii,['W_body/.,P',num2str(ii)])
      |             port_label('input', ii,['Xddot,P',num2str(ii)])
      |         else
      |             port_label('input', ii,['W_./body,P',num2str(ii)])
      |             port_label('output',ii,['Xddot,P',num2str(ii)])
      |         end
      |     end
      | end
  Multi port rigid body9 : Subsystem  mask(Multi-port rigid body (6nx6n)){m=1.219, Ig=[0.111172755531 0 0;0 0.111172755531 0;0 0 0.21942], OG=[0;0;0], n=2, numinv=1, OP1=[0;0;0], OP2=[0; 0; -0.09465], OP3=[0;0;0], OP4=[0;0;0], OP5=[0;0;0]}
      mask prompts: m "Mass (Kg)"; Ig "Inertia (at G, Kg m^2)"; OG "OG (3x1 vector, m)"; n "Number of ports"; numinv "Port to be inverted"; OP1 "OP1 (3x1 vector, m)"; OP2 "OP2 (3x1 vector, m)"; OP3 "OP3 (3x1 vector, m)"; OP4 "OP4 (3x1 vector, m)"; OP5 "OP5 (3x1 vector,m)"
      mask help:
      | 6nx6n dynamic model of a rigid body at n given points (ports) between wrenches applied at the n points (input) and acceleration twists at these points (output).
      |
      | 0: the reference point
      | G: the center of mass
      | Pi (i=1:n): the n given connection points (n<6).
      |
      | All parameters are expressed in the body frame.
      | Each parameter can be an uncertain parameter declared with "ureal"
      |
      | The 6x6 channel associated to one port can be inverted: then the input of this channel is the acceleration twist imposed at this point and the output is the wrench applied by this body.
      mask init:
      | MultiPortRigidBody
      mask Help: web('Docmultiportrigidbody.html')
      mask TypeOptions n: 1 | 2 | 3 | 4 | 5
      mask TypeOptions numinv: none | 1 | 2 | 3 | 4 | 5
      mask DialogControl ParameterGroupVar Prompt: Main parameters
      mask DialogControl port1 Prompt: Port #1
      mask DialogControl port2 Prompt: #2
      mask DialogControl port3 Prompt: #3
      mask DialogControl port4 Prompt: #4
      mask DialogControl port5 Prompt: #5
      mask Display:
      | disp('Multi-port\n rigid body\n (6nx6n)')
      | if n==1,
      |     if numinv-1==1,
      |         port_label('input', 1,'Xddot,P')
      |         port_label('output',1,'W_body/.,P')
      |     else
      |         port_label('input', 1,'W_./body,P')
      |         port_label('output',1,'Xddot,P')
      |     end
      | else
      |     for ii=1:n
      |         if numinv==ii+1,
      |             port_label('output',ii,['W_body/.,P',num2str(ii)])
      |             port_label('input', ii,['Xddot,P',num2str(ii)])
      |         else
      |             port_label('input', ii,['W_./body,P',num2str(ii)])
      |             port_label('output',ii,['Xddot,P',num2str(ii)])
      |         end
      |     end
      | end
  W_body : Outport
  Outport : Outport  Port=2
  wires:
  6x6 v-u_rotation9/1 -> Multi port rigid body3/2(W_./body,P2)
  Multi port rigid body7/1(W_body/.,P1) -> W_body/1
  Multi port rigid body6/1(W_body/.,P1) -> 6x6 v-u_rotation13/1
  Multi port rigid body8/2(Xddot,P2) -> 6x6 v-u_rotation4/1
  Multi port rigid body1/2(Xddot,P2) -> 6x6 v-u_rotation6/1
  Multi port rigid body4/1(W_body/.,P1) -> 6x6 v-u_rotation9/1
  Multi port rigid body3/1(W_body/.,P1) -> 6x6 v-u_rotation7/1
  Multi port rigid body8/1(W_body/.,P1) -> 6x6 v-u_rotation3/1
  6x6 v-u_rotation13/1 -> Multi port rigid body9/2(W_./body,P2)
  6x6 v-u_rotation4/1 -> Multi port rigid body1/1(Xddot,P1)
  6x6 v-u_rotation3/1 -> Multi port rigid body7/2(W_./body,P2)
  6x6 v-u_rotation5/1 -> Multi port rigid body8/2(W_./body,P2)
  6x6 v-u_rotation8/1 -> Multi port rigid body4/1(Xddot,P1)
  6x6 v-u_rotation6/1 -> Multi port rigid body3/1(Xddot,P1)
  Xddot/1 -> Multi port rigid body7/1(Xddot,P1)
  Multi port rigid body9/1(W_body/.,P1) -> 6x6 v-u_rotation11/1
  6x6 v-u_rotation12/1 -> Multi port rigid body6/1(Xddot,P1)
  Multi port rigid body7/2(Xddot,P2) -> 6x6 v-u_rotation2/1
  Multi port rigid body3/2(Xddot,P2) -> 6x6 v-u_rotation8/1
  6x6 v-u_rotation10/1 -> Multi port rigid body9/1(Xddot,P1)
  6x6 v-u_rotation7/1 -> Multi port rigid body1/2(W_./body,P2)
  6x6 v-u_rotation11/1 -> Multi port rigid body4/2(W_./body,P2)
  6x6 v-u_rotation2/1 -> Multi port rigid body8/1(Xddot,P1)
  Multi port rigid body9/2(Xddot,P2) -> 6x6 v-u_rotation12/1
  Multi port rigid body4/2(Xddot,P2) -> 6x6 v-u_rotation10/1
  Multi port rigid body1/1(W_body/.,P1) -> 6x6 v-u_rotation5/1
  Multi port rigid body6/2(Xddot,P2) -> Outport/1
  Inport/1 -> Multi port rigid body6/2(W_./body,P2)

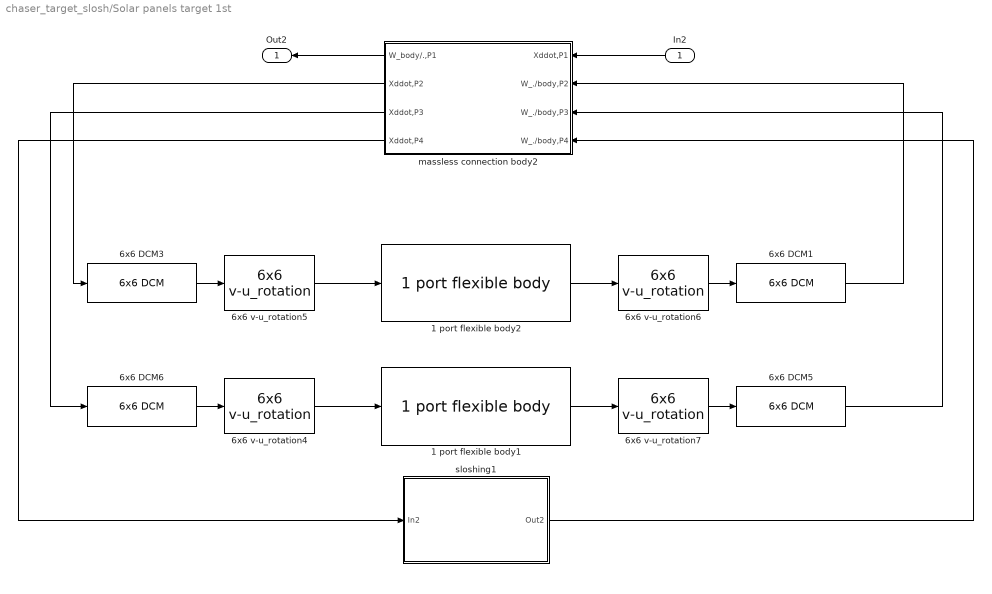
== system chaser_target_slosh/Solar panels target 1st ==
  In2 : Inport
  1 port flexible body1 : SDTlibV1/6 dof bodies/1 port flexible body  m=solar_panel_target_reduced_FEM.m  Ig=inertias_target  OG=r_PG_target  OP=[0;0;0]  n=6  xi=solar_panel_target_reduced_FEM.xi  w1=ureal('wntarget1',wn_target(1),'Percentage',20);  L11=solar_panel_target_reduced_FEM.L(1,1)  L12=solar_panel_target_reduced_FEM.L(1,2)  L13=solar_panel_target_reduced_FEM.L(1,3)  L14=solar_panel_target_reduced_FEM.L(1,4)  L15=solar_panel_target_reduced_FEM.L(1,5)  L16=solar_panel_target_reduced_FEM.L(1,6)  w2=wn_target(2)  L21=solar_panel_target_reduced_FEM.L(2,1)  L22=solar_panel_target_reduced_FEM.L(2,2)  L23=solar_panel_target_reduced_FEM.L(2,3)  L24=solar_panel_target_reduced_FEM.L(2,4)  L25=solar_panel_target_reduced_FEM.L(2,5)  L26=solar_panel_target_reduced_FEM.L(2,6)  w3=wn_target(3)  L31=solar_panel_target_reduced_FEM.L(3,1)  L32=solar_panel_target_reduced_FEM.L(3,2)  L33=solar_panel_target_reduced_FEM.L(3,3)  L34=solar_panel_target_reduced_FEM.L(3,4)  L35=solar_panel_target_reduced_FEM.L(3,5)  L36=solar_panel_target_reduced_FEM.L(3,6)  w4=wn_target(4)  L41=solar_panel_target_reduced_FEM.L(4,1)  L42=solar_panel_target_reduced_FEM.L(4,2)  L43=solar_panel_target_reduced_FEM.L(4,3)  L44=solar_panel_target_reduced_FEM.L(4,4)  L45=solar_panel_target_reduced_FEM.L(4,5)  L46=solar_panel_target_reduced_FEM.L(4,6)  w5=wn_target(5)  L51=solar_panel_target_reduced_FEM.L(5,1)  L52=solar_panel_target_reduced_FEM.L(5,2)  L53=solar_panel_target_reduced_FEM.L(5,3)  L54=solar_panel_target_reduced_FEM.L(5,4)  L55=solar_panel_target_reduced_FEM.L(5,5)  L56=solar_panel_target_reduced_FEM.L(5,6)  w6=wn_target(6)  L61=solar_panel_target_reduced_FEM.L(6,1)  L62=solar_panel_target_reduced_FEM.L(6,2)  L63=solar_panel_target_reduced_FEM.L(6,3)  L64=solar_panel_target_reduced_FEM.L(6,4)  L65=solar_panel_target_reduced_FEM.L(6,5)  L66=solar_panel_target_reduced_FEM.L(6,6)  w7=0  L71=0  L72=0  L73=0  L74=0  L75=0  L76=0  w8=0  L81=0  L82=0  L83=0  L84=0  L85=0  L86=0  w9=0  L91=0  L92=0  L93=0  L94=0  L95=0  L96=0  w10=0  L101=0  L102=0  L103=0  L104=0  L105=0  L106=0
      settings: SourceProductName=SDTlib
  1 port flexible body2 : SDTlibV1/6 dof bodies/1 port flexible body  m=solar_panel_target_reduced_FEM.m  Ig=inertias_target  OG=r_PG_target  OP=[0;0;0]  n=6  xi=solar_panel_target_reduced_FEM.xi  w1=ureal('wntarget1',wn_target(1),'Percentage',20);  L11=solar_panel_target_reduced_FEM.L(1,1)  L12=solar_panel_target_reduced_FEM.L(1,2)  L13=solar_panel_target_reduced_FEM.L(1,3)  L14=solar_panel_target_reduced_FEM.L(1,4)  L15=solar_panel_target_reduced_FEM.L(1,5)  L16=solar_panel_target_reduced_FEM.L(1,6)  w2=wn_target(2)  L21=solar_panel_target_reduced_FEM.L(2,1)  L22=solar_panel_target_reduced_FEM.L(2,2)  L23=solar_panel_target_reduced_FEM.L(2,3)  L24=solar_panel_target_reduced_FEM.L(2,4)  L25=solar_panel_target_reduced_FEM.L(2,5)  L26=solar_panel_target_reduced_FEM.L(2,6)  w3=wn_target(3)  L31=solar_panel_target_reduced_FEM.L(3,1)  L32=solar_panel_target_reduced_FEM.L(3,2)  L33=solar_panel_target_reduced_FEM.L(3,3)  L34=solar_panel_target_reduced_FEM.L(3,4)  L35=solar_panel_target_reduced_FEM.L(3,5)  L36=solar_panel_target_reduced_FEM.L(3,6)  w4=wn_target(4)  L41=solar_panel_target_reduced_FEM.L(4,1)  L42=solar_panel_target_reduced_FEM.L(4,2)  L43=solar_panel_target_reduced_FEM.L(4,3)  L44=solar_panel_target_reduced_FEM.L(4,4)  L45=solar_panel_target_reduced_FEM.L(4,5)  L46=solar_panel_target_reduced_FEM.L(4,6)  w5=wn_target(5)  L51=solar_panel_target_reduced_FEM.L(5,1)  L52=solar_panel_target_reduced_FEM.L(5,2)  L53=solar_panel_target_reduced_FEM.L(5,3)  L54=solar_panel_target_reduced_FEM.L(5,4)  L55=solar_panel_target_reduced_FEM.L(5,5)  L56=solar_panel_target_reduced_FEM.L(5,6)  w6=wn_target(6)  L61=solar_panel_target_reduced_FEM.L(6,1)  L62=solar_panel_target_reduced_FEM.L(6,2)  L63=solar_panel_target_reduced_FEM.L(6,3)  L64=solar_panel_target_reduced_FEM.L(6,4)  L65=solar_panel_target_reduced_FEM.L(6,5)  L66=solar_panel_target_reduced_FEM.L(6,6)  w7=0  L71=0  L72=0  L73=0  L74=0  L75=0  L76=0  w8=0  L81=0  L82=0  L83=0  L84=0  L85=0  L86=0  w9=0  L91=0  L92=0  L93=0  L94=0  L95=0  L96=0  w10=0  L101=0  L102=0  L103=0  L104=0  L105=0  L106=0
      settings: SourceProductName=SDTlib
  6x6 DCM1 : SDTlibV1/3//6 dof DCM/6x6 DCM  rot=chaser.solarpanel.R(:,:,1)  transp=off
      settings: SourceProductName=SDTlib
  6x6 DCM3 : SDTlibV1/3//6 dof DCM/6x6 DCM  rot=chaser.solarpanel.R(:,:,1)  transp=on
      settings: SourceProductName=SDTlib
  6x6 DCM5 : SDTlibV1/3//6 dof DCM/6x6 DCM  rot=chaser.solarpanel.R(:,:,2)  transp=off
      settings: SourceProductName=SDTlib
  6x6 DCM6 : SDTlibV1/3//6 dof DCM/6x6 DCM  rot=chaser.solarpanel.R(:,:,2)  transp=on
      settings: SourceProductName=SDTlib
  6x6 v-u_rotation4 : SDTlibV1/3//6 dof DCM/6x6 v-u_rotation  ra=[0;1;0]  theta=ureal('theta10',0,'Range',[-pi pi])  transp=on
      settings: SourceProductName=SDTlib
  6x6 v-u_rotation5 : SDTlibV1/3//6 dof DCM/6x6 v-u_rotation  ra=[0;1;0]  theta=ureal('theta9',0,'Range',[-pi pi])  transp=on
      settings: SourceProductName=SDTlib
  6x6 v-u_rotation6 : SDTlibV1/3//6 dof DCM/6x6 v-u_rotation  ra=[0;1;0]  theta=ureal('theta9',0,'Range',[-pi pi])  transp=off
      settings: SourceProductName=SDTlib
  6x6 v-u_rotation7 : SDTlibV1/3//6 dof DCM/6x6 v-u_rotation  ra=[0;1;0]  theta=ureal('theta10',0,'Range',[-pi pi])  transp=off
      settings: SourceProductName=SDTlib
  massless connection body2 : Subsystem  mask(Massless multi_port (6nx6n)){n=4, numinv=1, OP1=[0;0;0], OP2=chaser.solarpanel.location(:,1)*0.7, OP3=chaser.solarpanel.location(:,2)*0.7, OP4=[0;0;0], OP5=chaser.GNC.control.reaction_wheels.positions(:,4), OP6=[0;0;0], OP7=[0;0;0]}
      mask prompts: n "Number of ports"; numinv "Port (point) Pj: j="; OP1 "OP1 (3x1 vector, m)"; OP2 "OP2 (3x1 vector, m)"; OP3 "OP3 (3x1 vector, m)"; OP4 "OP4 (3x1 vector, m)"; OP5 "OP5 (3x1 vector,m)"; OP6 "OP6 (3x1 vector,m)"; OP7 "OP7 (3x1 vector,m)"
      mask help:
      | Massless body to transport wrenches and acceleration twists:
      | 6nx6n gain from:
      |  * the acceleration twist at one point Pj; i.e. the parent port,
      |  * the wrenches applied to this massless body at the n-1 points Pi (i=1,..n, except j); i.e. the child ports
      | to:
      |  * the wrench applied at point Pj by this massless body,
      |  * the accelaretion twists at the other n-1  points Pi (i=1,..n, except j).
      |
      | 0: the reference point
      | Pi (i=1:n): the n given connection points or ports (1<n<8).
      |
      | All parameters are expressed in the body frame.
      | Each parameter can be an uncertain parameter declared with "ureal"
      mask init:
      | MasslessConnectionBody
      mask Help: web('DocMassLessBody.html')
      mask TypeOptions n: 2 | 3 | 4 | 5 | 6 | 7
      mask TypeOptions numinv: 1 | 2 | 3 | 4 | 5 | 6 | 7
      mask DialogControl ParameterGroupVar Prompt: Main parameters
      mask DialogControl port1 Prompt: Port #1
      mask DialogControl port2 Prompt: #2
      mask DialogControl port3 Prompt: #3
      mask DialogControl port4 Prompt: #4
      mask DialogControl port5 Prompt: #5
      mask DialogControl port6 Prompt: #6
      mask DialogControl port7 Prompt: #7
      mask Display:
      | disp('Massless\n connection body\n (6nx6n)')
      | for ii=1:n+1
      |     if numinv==ii,
      |         port_label('output',ii,['W_body/.,P',num2str(ii)])
      |         port_label('input', ii,['Xddot,P',num2str(ii)])
      |     else
      |         port_label('input', ii,['W_./body,P',num2str(ii)])
      |         port_label('output',ii,['Xddot,P',num2str(ii)])
      |     end
      | end
  sloshing1 : Subsystem
  Out2 : Outport
  wires:
  massless connection body2/1(W_body/.,P1) -> Out2/1
  In2/1 -> massless connection body2/1(Xddot,P1)
  1 port flexible body2/1 -> 6x6 v-u_rotation6/1
  6x6 v-u_rotation5/1 -> 1 port flexible body2/1
  6x6 v-u_rotation6/1 -> 6x6 DCM1/1
  1 port flexible body1/1 -> 6x6 v-u_rotation7/1
  massless connection body2/2(Xddot,P2) -> 6x6 DCM3/1
  6x6 DCM1/1 -> massless connection body2/2(W_./body,P2)
  6x6 DCM3/1 -> 6x6 v-u_rotation5/1
  6x6 v-u_rotation7/1 -> 6x6 DCM5/1
  6x6 DCM5/1 -> massless connection body2/3(W_./body,P3)
  6x6 v-u_rotation4/1 -> 1 port flexible body1/1
  6x6 DCM6/1 -> 6x6 v-u_rotation4/1
  massless connection body2/3(Xddot,P3) -> 6x6 DCM6/1
  sloshing1/1(Out2) -> massless connection body2/4(W_./body,P4)
  massless connection body2/4(Xddot,P4) -> sloshing1/1(In2)
